simulink subsystem "controller_3dof"  (R2025b)
settings: Solver=VariableStepAuto  StartTime=0.0  StopTime=10.0  RelTol=1e-3
settings Model: Creator=schwmaxi  LastModifiedBy=schwmaxi

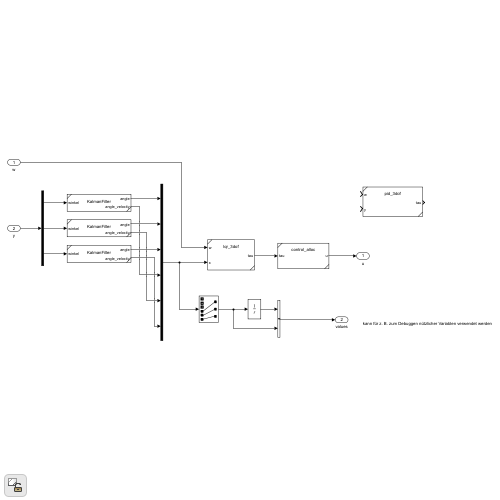
[thumbnail: Simulink's stored preview of the top-level diagram]
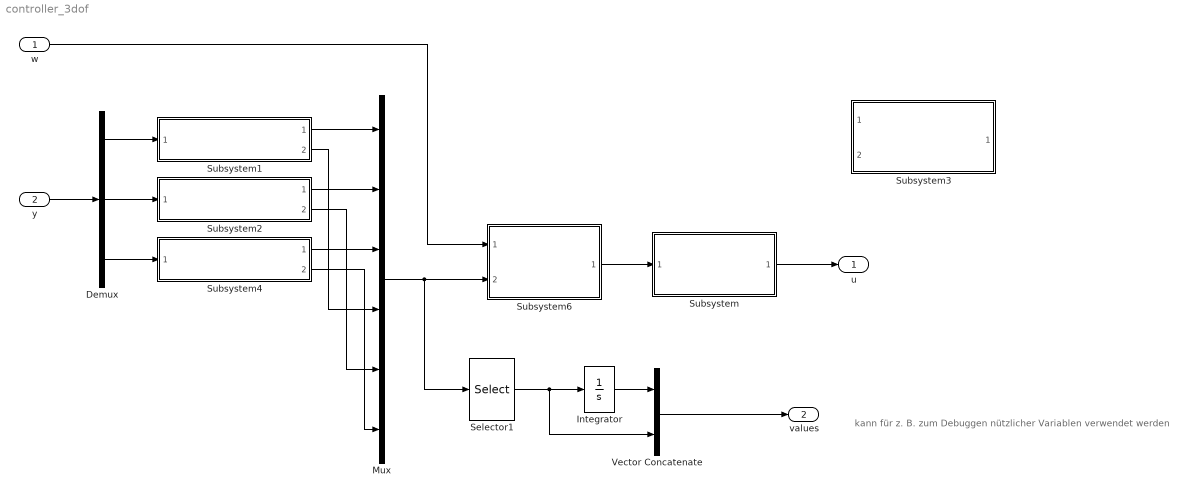
== system controller_3dof ==
  note: kann für z. B. zum Debuggen nützlicher Variablen verwendet werden
  w : Inport
  y : Inport  Port=2
  Demux : Demux  Outputs=3
  Integrator : Integrator
  Mux : Mux  Inputs=6
  Selector1 : Selector  InputPortWidth=6  IndexOptions=Index vector (dialog)  Indices=[4 5 6]  OutputSizes=1
  Subsystem : Subsystem  ReferencedSubsystem=control_alloc
  Subsystem1 : Subsystem  ReferencedSubsystem=KalmanFilter
  Subsystem2 : Subsystem  ReferencedSubsystem=KalmanFilter
  Subsystem3 : Subsystem  ReferencedSubsystem=pid_3dof
  Subsystem4 : Subsystem  ReferencedSubsystem=KalmanFilter
  Subsystem6 : Subsystem  ReferencedSubsystem=lqr_3dof
  Vector Concatenate : Concatenate
  u : Outport
  values : Outport  Port=2
  wires:
  Subsystem2/1 -> Mux/2
  Demux/3 -> Subsystem4/1
  Subsystem2/2 -> Mux/5
  Demux/2 -> Subsystem2/1
  y/1 -> Demux/1
  Subsystem4/1 -> Mux/3
  Subsystem4/2 -> Mux/6
  Selector1/1 -> Integrator/1, Vector Concatenate/2
  Integrator/1 -> Vector Concatenate/1
  Vector Concatenate/1 -> values/1
  Subsystem/1 -> u/1
  Demux/1 -> Subsystem1/1
  Subsystem1/1 -> Mux/1
  Subsystem1/2 -> Mux/4
  Subsystem6/1 -> Subsystem/1
  Mux/1 -> Selector1/1, Subsystem6/2
  w/1 -> Subsystem6/1
